simulink library "common_lib"  (Simulink 7.9)
settings: Solver=ode45  StartTime=0.0  StopTime=10.0  RelTol=1e-3
libraries: simulink x1
settings Model: Creator=fguerin  LastModifiedBy=klindqvi

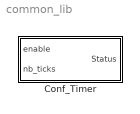
== system common_lib ==
  Conf_Timer : Subsystem

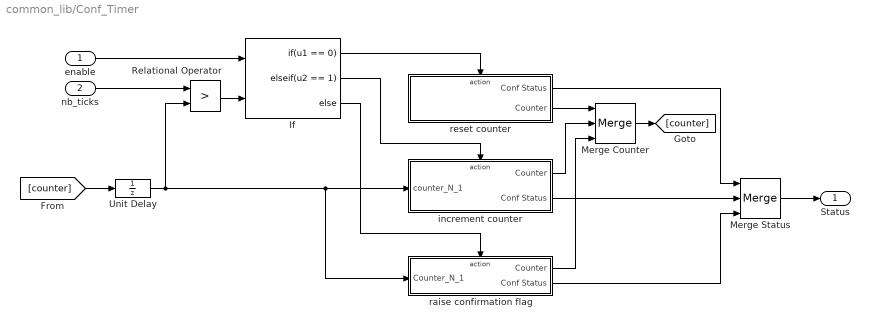
== system common_lib/Conf_Timer ==
  enable : Inport  OutMin=0  OutMax=1  OutDataTypeStr=boolean  PortDimensions=1  Interpolate=off
  nb_ticks : Inport  Port=2  OutMin=0  OutMax=65535  OutDataTypeStr=uint16  PortDimensions=1  Interpolate=off
  If : If  NumInputs=2  IfExpression=u1 == 0  ElseIfExpressions=u2 == 1
  Merge Counter : Merge  Inputs=3
  Merge Status : Merge  Inputs=3
  Relational Operator : RelationalOperator  Operator=>  OutDataTypeStr=boolean  InputSameDT=on
  Unit Delay : UnitDelay  SampleTime=-1
  increment counter : Subsystem  TreatAsAtomicUnit=on
  raise confirmation flag : Subsystem  TreatAsAtomicUnit=on
  reset counter : Subsystem  TreatAsAtomicUnit=on
  Status : Outport  OutMin=0  OutMax=1  OutDataTypeStr=boolean  PortDimensions=1
  wires:
  If/3 -> raise confirmation flag/Action
  reset counter/2(Counter) -> Merge Counter/1
  increment counter/1(Counter) -> Merge Counter/2
  If/1 -> reset counter/Action
  enable/1 -> If/1
  reset counter/1(Conf Status) -> Merge Status/1
  increment counter/2(Conf Status) -> Merge Status/2
  raise confirmation flag/2(Conf Status) -> Merge Status/3
  Merge Counter/1 -> [counter]
  Merge Status/1 -> Status/1
  [counter] -> Unit Delay/1
  nb_ticks/1 -> Relational Operator/1
  Relational Operator/1 -> If/2
  Unit Delay/1 -> Relational Operator/2, increment counter/1(counter_N_1), raise confirmation flag/1(Counter_N_1)
  If/2 -> increment counter/Action
  raise confirmation flag/1(Counter) -> Merge Counter/3

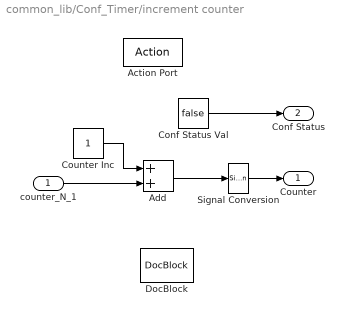
== system common_lib/Conf_Timer/increment counter ==
  counter_N_1 : Inport
  Action Port : ActionPort  PropagateVarSize=During execution
  Add : Sum  SaturateOnIntegerOverflow=on  InputSameDT=on
      settings: AttributesFormatString=Saturation:%<SaturateOnIntegerOverflow>
  Conf Status Val : Constant  Value=false  OutDataTypeStr=Inherit: Inherit via back propagation  SampleTime=-1
  Counter Inc : Constant  OutDataTypeStr=Inherit: Inherit via back propagation  SampleTime=-1
  DocBlock : simulink/Model-Wide Utilities/DocBlock  DocumentType=Text
      content=|
      | Derived Low Level Requirement:
      | The counter is saturated to avoid an integer overflow that would lead to a reset of the confirmation flag.
  Signal Conversion : SignalConversion  ConversionOutput=Contiguous copy
  Counter : Outport  InitialOutput=0
  Conf Status : Outport  Port=2  InitialOutput=0
  wires:
  Counter Inc/1 -> Add/1
  Conf Status Val/1 -> Conf Status/1
  Add/1 -> Signal Conversion/1
  counter_N_1/1 -> Add/2
  Signal Conversion/1 -> Counter/1

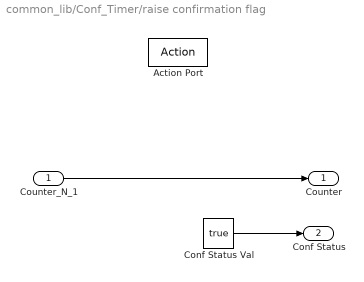
== system common_lib/Conf_Timer/raise confirmation flag ==
  Counter_N_1 : Inport
  Action Port : ActionPort  PropagateVarSize=During execution
  Conf Status Val : Constant  Value=true  OutDataTypeStr=Inherit: Inherit via back propagation  SampleTime=-1
  Counter : Outport  InitialOutput=0
  Conf Status : Outport  Port=2  InitialOutput=1
  wires:
  Conf Status Val/1 -> Conf Status/1
  Counter_N_1/1 -> Counter/1

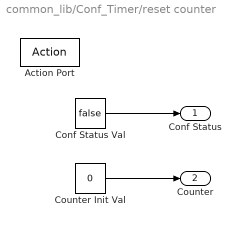
== system common_lib/Conf_Timer/reset counter ==
  Action Port : ActionPort  PropagateVarSize=During execution
  Conf Status Val : Constant  Value=false  OutDataTypeStr=Inherit: Inherit via back propagation  SampleTime=-1
  Counter Init Val : Constant  Value=0  OutDataTypeStr=Inherit: Inherit via back propagation  SampleTime=-1
  Conf Status : Outport  InitialOutput=0
  Counter : Outport  Port=2  InitialOutput=0
  wires:
  Counter Init Val/1 -> Counter/1
  Conf Status Val/1 -> Conf Status/1
